simulink model "sim10_rs"  (R2015b)
settings: Solver=VariableStepAuto  StartTime=0.0  StopTime=10.0  RelTol=1e-3
values from neighbouring files (symbols this model uses):
  dy_inicial = 0    [Lab2.m]
  k1 = 1/yl    (= 10)    [Lab2.m]    (also in u_valor.m = 1/yl)
  k2 = sqrt(2*k1)    [Lab2.m]    (also in u_valor.m)
  y_inicial = 1    [Lab2.m]
settings Model: Creator=Alice  LastModifiedBy=Alice

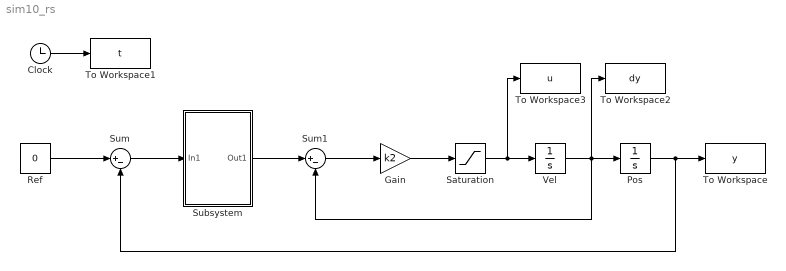
== system sim10_rs ==
  Clock : Clock
  Gain : Gain  Gain=k2
  Pos : Integrator  InitialCondition=y_inicial
  Ref : Constant  Value=0
  Saturation : Saturate  UpperLimit=1  LowerLimit=-1
  Subsystem : Subsystem
  Sum : Sum  Inputs=|+-
  Sum1 : Sum  Inputs=|+-
  To Workspace : ToWorkspace  VariableName=y  SampleTime=0.1
  To Workspace1 : ToWorkspace  VariableName=t  SampleTime=0.1
  To Workspace2 : ToWorkspace  VariableName=dy  SampleTime=0.1
  To Workspace3 : ToWorkspace  VariableName=u  SampleTime=0.1
  Vel : Integrator  InitialCondition=dy_inicial
  wires:
  Ref/1 -> Sum/1
  Sum/1 -> Subsystem/1(In1)
  Subsystem/1(Out1) -> Sum1/1
  Sum1/1 -> Gain/1
  Gain/1 -> Saturation/1
  Saturation/1 -> To Workspace3/1, Vel/1
  Vel/1 -> To Workspace2/1, Sum1/2, Pos/1
  Pos/1 -> To Workspace/1, Sum/2
  Clock/1 -> To Workspace1/1

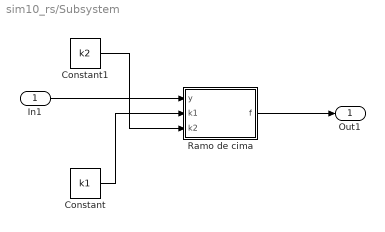
== system sim10_rs/Subsystem ==
  In1 : Inport
  Constant : Constant  Value=k1
  Constant1 : Constant  Value=k2
  Ramo de cima : MATLAB Function  TreatAsAtomicUnit=on
  Out1 : Outport
  wires:
  In1/1 -> Ramo de cima/1(y)
  Constant/1 -> Ramo de cima/2(k1)
  Constant1/1 -> Ramo de cima/3(k2)
  Ramo de cima/1(f) -> Out1/1

== matlab function sim10_rs/Subsystem/Ramo de cima ==
  data: y input; k1 input; f output; k2 input
function f = fcn(y,k1,k2)

f=(k1/k2)*(y);

end
